simulink subsystem "Dinamika"  (R2024b)
settings: Solver=VariableStepAuto  StartTime=0.0  StopTime=10.0  RelTol=1e-3
undefined symbols (not defined in the file or in its folder): c, J, L, M, R
settings Model: Creator=Asus  LastModifiedBy=Asus

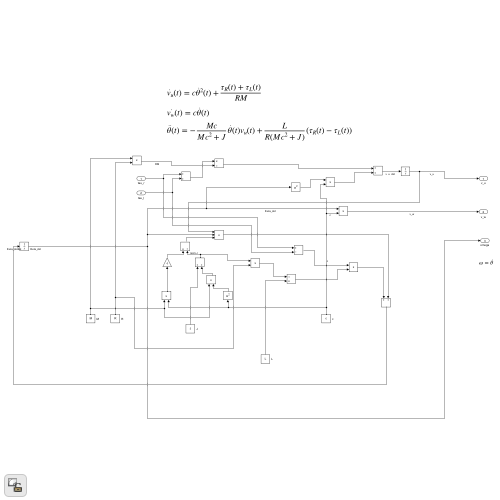
[thumbnail: Simulink's stored preview of the top-level diagram]
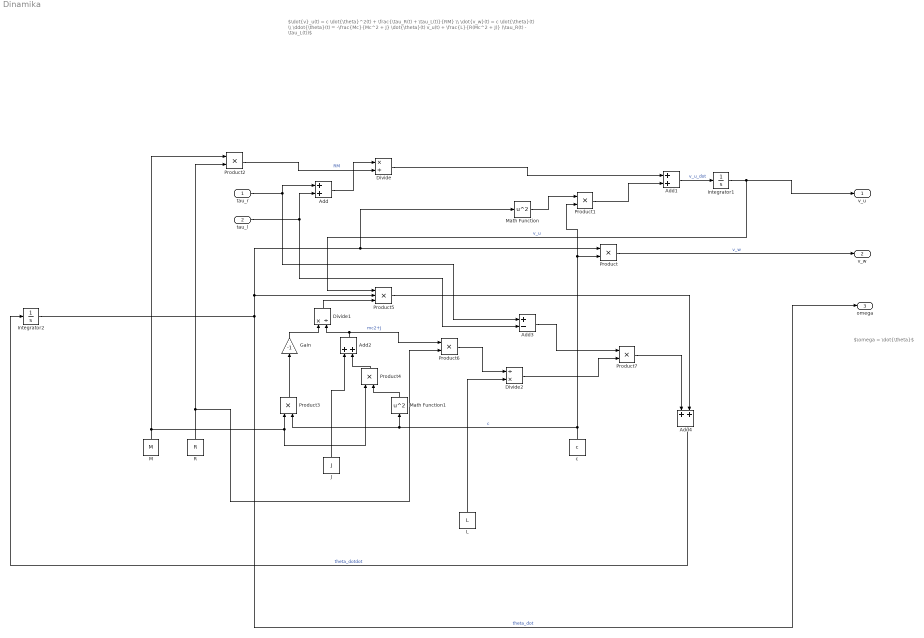
== system Dinamika ==
  note: $\omega = \dot{\theta}$
  note: $\dot{v}_u(t) = c \dot{\theta}^2(t) + \frac{\tau_R(t) + \tau_L(t)}{RM} \\ \dot{v_w}(t) = c \dot{\theta}(t) \\ \ddot{\theta}(t) = -\frac{Mc}{Mc^2 + J} \dot{\theta}(t) v_u(t) + \frac{L}{R(Mc^2 + J)} (\tau_R(t) - \tau_L(t))$
  tau_r : Inport
  tau_l : Inport  Port=2
  Add{,1..2,4} (4 alike) : Sum
  Add3 : Sum  Inputs=+-
  Divide : Product  Inputs=*/
  Divide1 : Product  Inputs=*/
  Divide2 : Product  Inputs=/*
  Gain : Gain  Gain=-1
  Integrator1 : Integrator
  Integrator2 : Integrator
  J : Constant  Value=J
  L : Constant  Value=L
  M : Constant  Value=M
  Math Function : Math  Operator=square
  Math Function1 : Math  Operator=square
  Product{,1..4,6..7} (7 alike) : Product
  Product5 : Product  Inputs=3
  R : Constant  Value=R
  c : Constant  Value=c
  v_u : Outport
  v_w : Outport  Port=2
  omega : Outport  Port=3
  wires:
  c/1 -> Product1/2, Product/2, Math Function1/1, Product3/2  "c"
  Product/1 -> v_w/1  "v_w"
  Math Function/1 -> Product1/1
  Product1/1 -> Add1/2
  R/1 -> Product6/2, Product2/2
  M/1 -> Product2/1, Product3/1, Product4/1
  Product2/1 -> Divide/2  "RM"
  tau_r/1 -> Add3/1, Add/1
  tau_l/1 -> Add/2, Add3/2
  Add/1 -> Divide/1
  Divide/1 -> Add1/1
  Add1/1 -> Integrator1/1  "v_u_dot"
  Integrator1/1 -> v_u/1, Product5/1  "v_u"
  Add4/1 -> Integrator2/1  "theta_dotdot"
  Math Function1/1 -> Product4/2
  Product4/1 -> Add2/2
  J/1 -> Add2/1
  Product3/1 -> Gain/1
  Gain/1 -> Divide1/1
  Add2/1 -> Divide1/2, Product6/1  "mc2+J"
  Divide1/1 -> Product5/3
  Integrator2/1 -> omega/1, Product5/2, Math Function/1, Product/1  "theta_dot"
  Product6/1 -> Divide2/1
  L/1 -> Divide2/2
  Divide2/1 -> Product7/2
  Add3/1 -> Product7/1
  Product7/1 -> Add4/1
  Product5/1 -> Add4/2
